simulink model "sample_model_2"  (R2023a)
settings: Solver=FixedStepAuto  StartTime=0.0  StopTime=10.0  RelTol=1e-3
libraries: androiduilib x3, androidsensorlib x2
settings Model: Creator=ragha  LastModifiedBy=Shesh
settings OptimizationCC: EnhancedBackFolding=on  PassReuseOutputArgsAs=Individual arguments  ZeroExternalMemoryAtStartup=off  ZeroInternalMemoryAtStartup=off  MaxStackSize=64  OptimizeBlockOrder=speed  DifferentSizesBufferReuse=on  OptimizationCustomize=off  EfficientTunableParamExpr=on
settings DebuggingCC: ParameterTunabilityLossMsg=error
settings HardwareCC: ProdBitPerPointer=32  ProdBitPerSizeT=32  ProdBitPerPtrDiffT=32  ProdLargestAtomicInteger=Long  ProdLargestAtomicFloat=Double  ProdWordSize=32  ProdHWDeviceType=ARM Compatible->ARM Cortex
settings SFSimCC: MATLABDynamicMemAlloc=off
settings RTWCC: Description=Embedded Coder  SystemTargetFile=ert.tlc  HardwareBoard=Android Device  TLCOptions="-aInlineSetEventsForThisBaseRateFcn=TLC_FALSE -aSuppressMultiTaskScheduler=TLC_FALSE  -aRateBasedStepFcn=0"  TemplateMakefile=ert_default_tmf  RTWVerbose=off  Toolchain=Android SDK/NDK Tools
settings CodeAppCC: ForceParamTrailComments=on  IgnoreCustomStorageClasses=off  OperatorAnnotations=on  SimulinkDataObjDesc=on  SFDataObjDesc=on  InsertBlockDesc=on

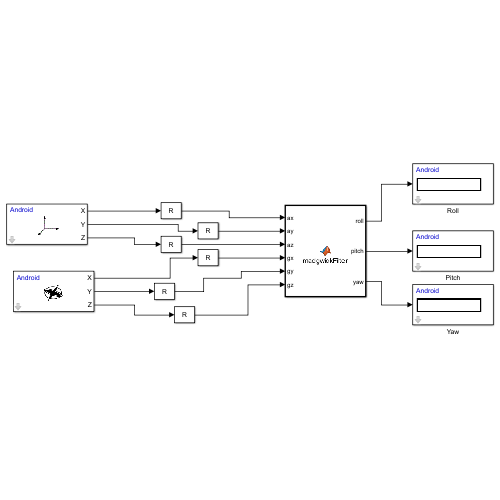
[thumbnail: Simulink's stored preview of the top-level diagram]
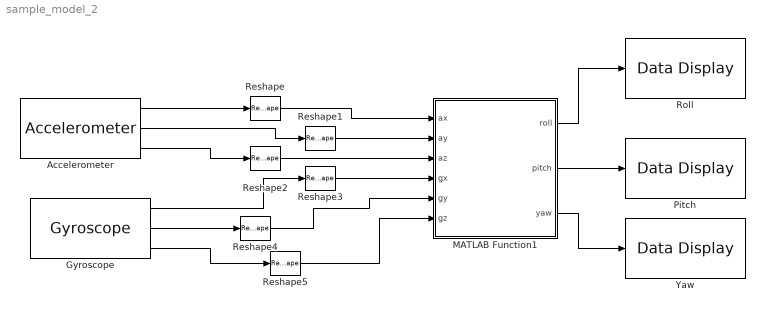
== system sample_model_2 ==
  Accelerometer : androidsensorlib/Accelerometer  OutputVector=off  SampleTime=0.5  BlockPlatform=Android
  Gyroscope : androidsensorlib/Gyroscope  OutputVector=off  SampleTime=0.5  BlockPlatform=Android
  MATLAB Function1 : MATLAB Function  TreatAsAtomicUnit=on
  Pitch : androiduilib/Data Display  DataDisplayId=sample_model_2/Pitch  Format=Float  Precision=6  SimulateUsing=Code generation  blockPlatform=Android
  Reshape{,1..5} (6 alike) : Reshape  OutputDimensionality=Customize  OutputDimensions=[1]
  Roll : androiduilib/Data Display  DataDisplayId=sample_model_2/Roll  Format=Float  Precision=6  SimulateUsing=Code generation  blockPlatform=Android
  Yaw : androiduilib/Data Display  DataDisplayId=sample_model_2/Yaw  Format=Float  Precision=6  SimulateUsing=Code generation  blockPlatform=Android
  wires:
  MATLAB Function1/1(roll) -> Roll/1
  MATLAB Function1/3(yaw) -> Yaw/1
  MATLAB Function1/2(pitch) -> Pitch/1
  Accelerometer/1 -> Reshape/1
  Accelerometer/2 -> Reshape1/1
  Accelerometer/3 -> Reshape2/1
  Gyroscope/1 -> Reshape3/1
  Gyroscope/2 -> Reshape4/1
  Gyroscope/3 -> Reshape5/1
  Reshape/1 -> MATLAB Function1/1(ax)
  Reshape1/1 -> MATLAB Function1/2(ay)
  Reshape2/1 -> MATLAB Function1/3(az)
  Reshape3/1 -> MATLAB Function1/4(gx)
  Reshape4/1 -> MATLAB Function1/5(gy)
  Reshape5/1 -> MATLAB Function1/6(gz)

== matlab function sample_model_2/MATLAB Function1 ==
  data: ax input; roll output; ay input; az input; gx input; gy input; gz input; pitch output; yaw output
function [roll, pitch, yaw] = madgwickFilter(ax, ay, az, gx, gy, gz)  
    deltaT = 0.1;
    persistent q_est;
    beta = 0.01;
    if isempty(q_est)
        q_est = [1; 0; 0; 0]; % Initial quaternion estimate
    end
    
    % Normalize accelerometer data
    a_norm = [ax; ay; az] / norm([ax, ay, az]);
    
    % Compute gradient and update quaternion using sensor data
    q_est_prev = q_est;
    q_w = [0; gx; gy; gz] * (deltaT / 2);
    
    gradient = computeGradient(q_est_prev, a_norm, beta);
    q_est_dot = q_w - gradient * deltaT;
    q_est = double(q_est_prev + q_est_dot * deltaT);
    jj = quatnormalize(q_est'); % Normalize quaternion
    
    % Convert quaternion to Euler angles
    
    [yaw,pitch,roll] = myQuat2Angle(jj');
    
    yaw = rad2deg(yaw);
    pitch = rad2deg(pitch);
    roll = rad2deg(roll);
end

function gradient = computeGradient(q_est, a_norm, beta)
    F_g = 2 * [q_est(2)*q_est(4) - q_est(1)*q_est(3) - a_norm(1);
               q_est(1)*q_est(2) + q_est(3)*q_est(4) - a_norm(2);
               0.5 - q_est(2)^2 - q_est(3)^2 - a_norm(3)];
           
    J_g = [-2*q_est(3), 2*q_est(4), -2*q_est(1), 2*q_est(2);
            2*q_est(2), 2*q_est(1), 2*q_est(4), 2*q_est(3);
            0, -4*q_est(2), -4*q_est(3), 0];
        
    gradient = J_g' * F_g;
    gradient = gradient * beta;
end
function [yaw, pitch, roll] = myQuat2Angle(q)
    % Ensure the quaternion is normalized
    q = q / norm(q);

    % Extract quaternion components
    w = q(1);
    x = q(2);
    y = q(3);
    z = q(4);

    % Compute Euler angles (yaw, pitch, roll) using 'ZYX' rotation sequence
    sinr_cosp = 2 * (w * x + y * z);
    cosr_cosp = 1 - 2 * (x^2 + y^2);
    roll = atan2(sinr_cosp, cosr_cosp);

    sinp = 2 * (w * y - z * x);
    if abs(sinp) >= 1
        pitch = sign(sinp) * pi / 2; % Use +/-90 degrees if out of range
    else
        pitch = asin(sinp);
    end

    siny_cosp = 2 * (w * z + x * y);
    cosy_cosp = 1 - 2 * (y^2 + z^2);
    yaw = atan2(siny_cosp, cosy_cosp);
    
    % Convert radians to degrees
    yaw = rad2deg(yaw);
    pitch = rad2deg(pitch);
    roll = rad2deg(roll);
end
